simulink model "first"  (R2018b)
settings: Solver=VariableStepAuto  StartTime=0.0  StopTime=10.0  MaxStep=0.01  RelTol=1e-3
settings Model: Creator=kekos  LastModifiedBy=kekos

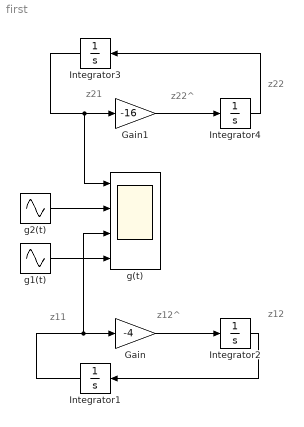
== system first ==
  note: z11
  note: z12^
  note: z12
  note: z21
  note: z22^
  note: z22
  Gain : Gain  Gain=-4
  Gain1 : Gain  Gain=-16
  Integrator1 : Integrator
  Integrator2 : Integrator  InitialCondition=10
  Integrator3 : Integrator
  Integrator4 : Integrator  InitialCondition=36
  g(t) : Scope  NumInputPorts=4
  g1(t) : Sin  Amplitude=5  Frequency=2  SampleTime=0
  g2(t) : Sin  Amplitude=9  Frequency=4  SampleTime=0
  wires:
  Gain/1 -> Integrator2/1
  Integrator2/1 -> Integrator1/1
  Integrator1/1 -> g(t)/3, Gain/1
  g1(t)/1 -> g(t)/4
  g2(t)/1 -> g(t)/2
  Gain1/1 -> Integrator4/1
  Integrator3/1 -> g(t)/1, Gain1/1
  Integrator4/1 -> Integrator3/1
